simulink library "rvs"  (R2016a)
settings: Solver=ode45  StartTime=0.0  StopTime=10.0  RelTol=1e-3
libraries: simulink x3
settings Model: Creator=Arthur  LastModifiedBy=arthur
settings DataIOCC: LimitDataPoints=on  SaveFormat=Array
settings DebuggingCC: SolverPrmCheckMsg=warning
settings HardwareCC: ProdBitPerPointer=32  ProdLargestAtomicFloat=None  ProdIntDivRoundTo=Undefined  ProdEndianess=Unspecified  ProdWordSize=32  ProdHWDeviceType=32-bit Generic
settings ModelReferenceCC: PropagateSignalLabelsOutOfModel=off
settings ConfigComp: CovModelRefEnable=Off  CovSFcnEnable=off

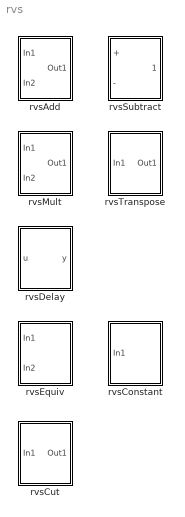
== system rvs ==
  rvsAdd : Subsystem  TreatAsAtomicUnit=on  mask(rvsAdd){}
      mask help: Add two signals
      mask Display: disp('+')
  rvsConstant : Subsystem  TreatAsAtomicUnit=on  mask(rvsConstant){}
      mask help: Require that the input signal must be constant
      mask Display: disp('? Const')
  rvsCut : Subsystem  TreatAsAtomicUnit=on  mask(rvsCut){}
      mask help: Direct pass through of signal from input to output but ignored by prover, so cuts off all static analysis information.
      mask Display: disp('Cut')
  rvsDelay : Subsystem  TreatAsAtomicUnit=on  mask(rvsDelay){xInit=[0]}
      mask prompts: xInit "Initial state"
      mask help: Unit delay.
      mask Display: disp('1\n--\nz')
  rvsEquiv : Subsystem  TreatAsAtomicUnit=on  mask(rvsEquiv){tol=1e-9, nIgnoreSteps=1}
      mask prompts: tol "Equality tolerance"; nIgnoreSteps "Initial steps to ignore"
      mask help: Test equivalence between two input signals.
      mask Display: disp('?==')
  rvsMult : Subsystem  TreatAsAtomicUnit=on  mask(rvsMult){}
      mask help: Matrix multiplication of two input signals.
      mask Display: disp('x')
  rvsSubtract : Subsystem  TreatAsAtomicUnit=on  mask(rvsSubtract){}
      mask help: Subtract two signals
  rvsTranspose : Subsystem  TreatAsAtomicUnit=on  mask(rvsTranspose){}
      mask help: Direct pass through of signal from input to output but ignored by prover, so cuts off all static analysis information.
      mask Display: disp('     T\nM')

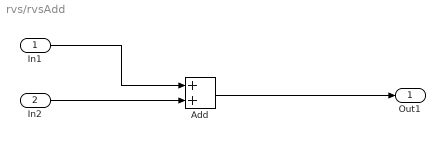
== system rvs/rvsAdd ==
  In1 : Inport
  In2 : Inport  Port=2
  Add : Sum
  Out1 : Outport
  wires:
  Add/1 -> Out1/1
  In2/1 -> Add/2
  In1/1 -> Add/1

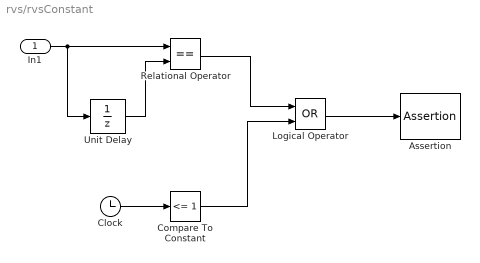
== system rvs/rvsConstant ==
  In1 : Inport
  Assertion : Assertion
  Clock : Clock
  Compare To Constant : simulink/Logic and Bit Operations/Compare To Constant  relop=<=  const=1  OutDataTypeStr=boolean
  Logical Operator : Logic  Operator=OR  AllPortsSameDT=off  OutDataTypeStr=boolean
  Relational Operator : RelationalOperator  Operator===  OutDataTypeStr=boolean
  Unit Delay : UnitDelay  SampleTime=-1
  wires:
  Compare To Constant/1 -> Logical Operator/2
  Clock/1 -> Compare To Constant/1
  Relational Operator/1 -> Logical Operator/1
  Logical Operator/1 -> Assertion/1
  Unit Delay/1 -> Relational Operator/2
  In1/1 -> Relational Operator/1, Unit Delay/1

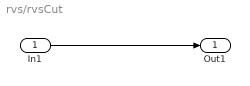
== system rvs/rvsCut ==
  In1 : Inport
  Out1 : Outport
  wires:
  In1/1 -> Out1/1

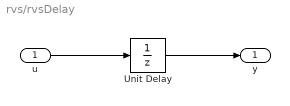
== system rvs/rvsDelay ==
  u : Inport
  Unit Delay : UnitDelay  InitialCondition=xInit  SampleTime=-1
  y : Outport
  wires:
  u/1 -> Unit Delay/1
  Unit Delay/1 -> y/1

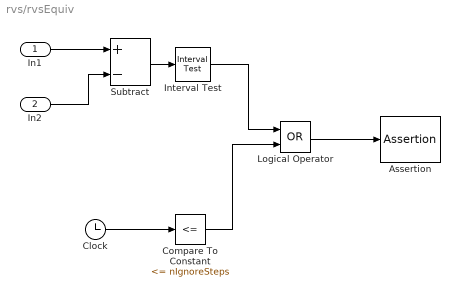
== system rvs/rvsEquiv ==
  In1 : Inport
  In2 : Inport  Port=2
  Assertion : Assertion
  Clock : Clock
  Compare To Constant : simulink/Logic and Bit Operations/Compare To Constant  relop=<=  const=nIgnoreSteps  OutDataTypeStr=boolean
  Interval Test : simulink/Logic and Bit Operations/Interval Test  IntervalClosedRight=on  uplimit=tol  IntervalClosedLeft=on  lowlimit=-tol  OutDataTypeStr=boolean
  Logical Operator : Logic  Operator=OR  AllPortsSameDT=off  OutDataTypeStr=boolean
  Subtract : Sum  Inputs=+-
  wires:
  Clock/1 -> Compare To Constant/1
  Interval Test/1 -> Logical Operator/1
  Logical Operator/1 -> Assertion/1
  Compare To Constant/1 -> Logical Operator/2
  Subtract/1 -> Interval Test/1
  In1/1 -> Subtract/1
  In2/1 -> Subtract/2

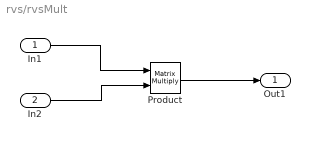
== system rvs/rvsMult ==
  In1 : Inport
  In2 : Inport  Port=2
  Product : Product  Multiplication=Matrix(*)
  Out1 : Outport
  wires:
  Product/1 -> Out1/1
  In2/1 -> Product/2
  In1/1 -> Product/1

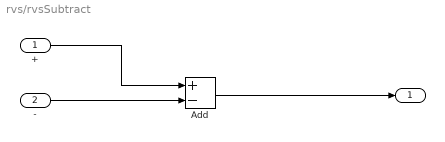
== system rvs/rvsSubtract ==
  + : Inport
  - : Inport  Port=2
  Add : Sum  Inputs=+-
  " " : Outport
  wires:
  Add/1 -> " "/1
  -/1 -> Add/2
  +/1 -> Add/1

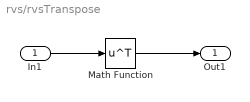
== system rvs/rvsTranspose ==
  In1 : Inport
  Math Function : Math  Operator=transpose  SaturateOnIntegerOverflow=on
  Out1 : Outport
  wires:
  In1/1 -> Math Function/1
  Math Function/1 -> Out1/1
